simulink model "Sim"  (R2025b)
settings: Solver=FixedStepAuto  StartTime=0.0  StopTime=15724800  FixedStep=300  RelTol=1e-3
values from neighbouring files (symbols this model uses):
  a = 3.5    [Regelung.m]
  b = -0.1    [Regelung.m]
  C = 5.0 * 10^7    (= 50000000)    [Regelung.m]
  eta = 0.20    (= 0.2)    [Regelung.m]
  R = 0.014    [Regelung.m]
settings Model: Creator=Mrhkf  LastModifiedBy=Mrhkf

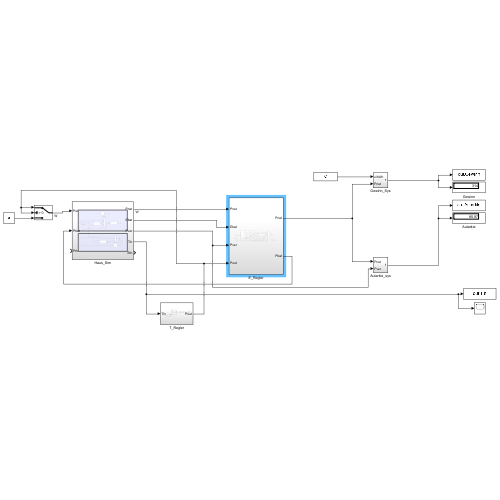
[thumbnail: Simulink's stored preview of the top-level diagram]
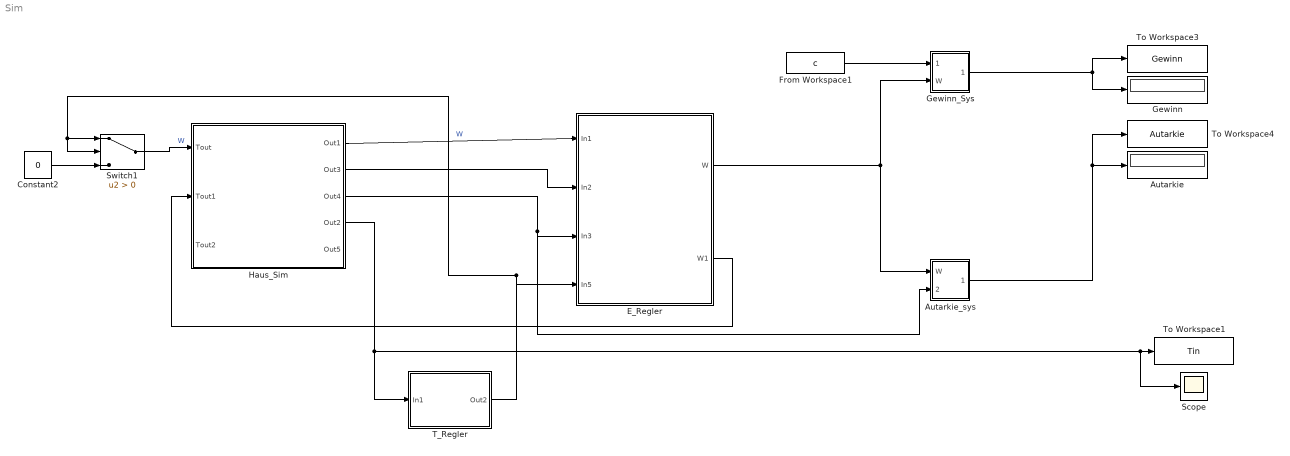
== system Sim ==
  Autarkie : Display
  Autarkie_sys : Subsystem
  Constant2 : Constant  Value=0
  E_Regler : Subsystem
  From Workspace1 : FromWorkspace  VariableName=c  SampleTime=-1  Interpolate=off  OutputAfterFinalValue=Holding final value
  Gewinn : Display
  Gewinn_Sys : Subsystem
  Haus_Sim : Subsystem
  Scope : Scope
      settings: ActiveDisplayYMinimum=17.325726119356677  ActiveDisplayYMaximum=22.113647259135355  DataLoggingVariableName=ScopeData8
  Switch1 : Switch  Criteria=u2 > Threshold  SaturateOnIntegerOverflow=off  InputSameDT=off
  T_Regler : Subsystem
  To Workspace1 : ToWorkspace  VariableName=Tin  SaveFormat=Timeseries  SampleTime=-1
  To Workspace3 : ToWorkspace  VariableName=Gewinn  SaveFormat=Timeseries  SampleTime=-1
  To Workspace4 : ToWorkspace  VariableName=Autarkie  SaveFormat=Timeseries  SampleTime=-1
  wires:
  Switch1/1 -> Haus_Sim/1(Tout)  "W"
  Constant2/1 -> Switch1/3
  Autarkie_sys/1(Out1) -> Autarkie/1, To Workspace4/1
  Gewinn_Sys/1(Out1) -> To Workspace3/1, Gewinn/1
  T_Regler/1(Out2) -> E_Regler/4(In5), Switch1/2, Switch1/1
  Haus_Sim/4(Out2) -> T_Regler/1(In1), Scope/1, To Workspace1/1
  Haus_Sim/3(Out4) -> Autarkie_sys/2(In2), E_Regler/3(In3)
  Haus_Sim/2(Out3) -> E_Regler/2(In2)
  Haus_Sim/1(Out1) -> E_Regler/1(In1)  "W"
  E_Regler/1(W) -> Gewinn_Sys/2(W), Autarkie_sys/1(W)
  From Workspace1/1 -> Gewinn_Sys/1(W1)
  E_Regler/2(W1) -> Haus_Sim/2(Tout1)

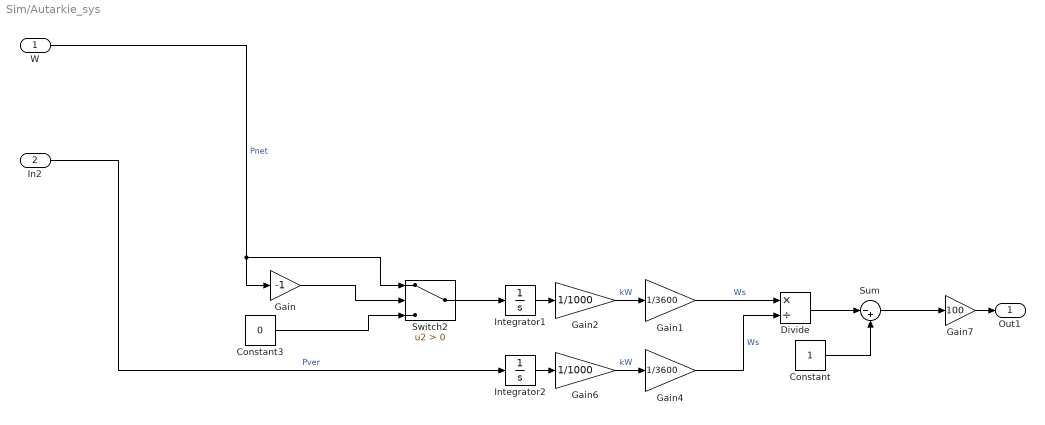
== system Sim/Autarkie_sys ==
  W : Inport
  In2 : Inport  Port=2
  Constant : Constant
  Constant3 : Constant  Value=0
  Divide : Product  Inputs=*/
  Gain : Gain  Gain=-1
  Gain1 : Gain  Gain=1/3600
  Gain2 : Gain  Gain=1/1000
  Gain4 : Gain  Gain=1/3600
  Gain6 : Gain  Gain=1/1000
  Gain7 : Gain  Gain=100
  Integrator1 : Integrator
  Integrator2 : Integrator
  Sum : Sum  Inputs=|-+
  Switch2 : Switch  Criteria=u2 > Threshold  SaturateOnIntegerOverflow=off  InputSameDT=off
  Out1 : Outport
  wires:
  Divide/1 -> Sum/1
  Switch2/1 -> Integrator1/1
  Integrator2/1 -> Gain6/1
  W/1 -> Gain/1, Switch2/1  "Pnet"
  Gain2/1 -> Gain1/1  "kW"
  Gain4/1 -> Divide/2  "Ws"
  Gain1/1 -> Divide/1  "Ws"
  Constant/1 -> Sum/2
  Integrator1/1 -> Gain2/1
  Sum/1 -> Gain7/1
  Gain6/1 -> Gain4/1  "kW"
  Constant3/1 -> Switch2/3
  Gain/1 -> Switch2/2
  Gain7/1 -> Out1/1
  In2/1 -> Integrator2/1  "Pver"

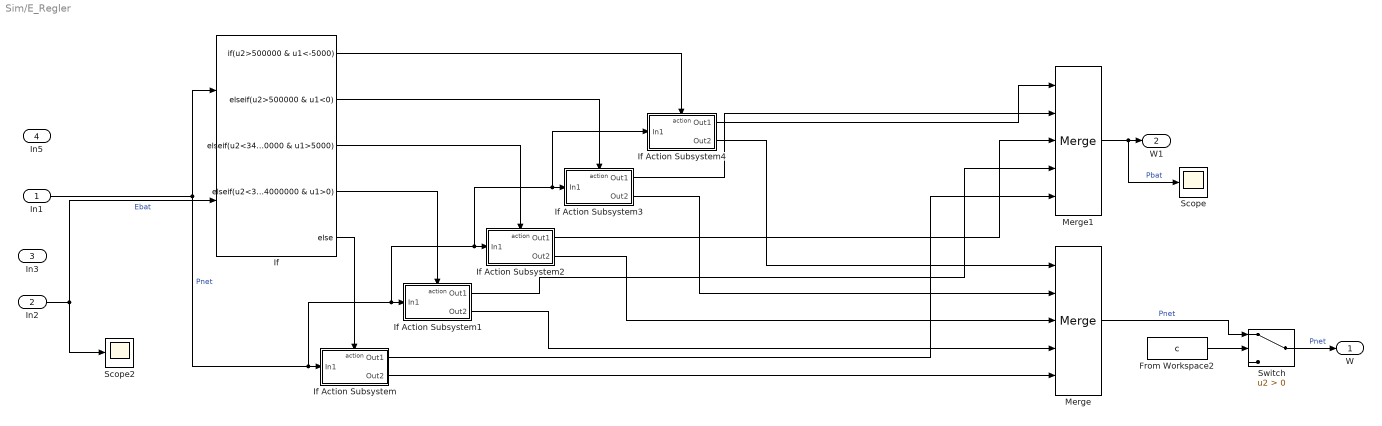
== system Sim/E_Regler ==
  In1 : Inport
  In2 : Inport  Port=2
  In3 : Inport  Port=3
  In5 : Inport  Port=4
  From Workspace2 : FromWorkspace  VariableName=c  SampleTime=-1  Interpolate=off  OutputAfterFinalValue=Holding final value
  If : If  NumInputs=2  IfExpression=u2>500000 & u1<-5000  ElseIfExpressions=u2>500000 & u1<0,u2<34000000 & u1>5000,u2<34000000 & u1>0
  If Action Subsystem : Subsystem  TreatAsAtomicUnit=on
  If Action Subsystem1 : Subsystem  TreatAsAtomicUnit=on
  If Action Subsystem2 : Subsystem  TreatAsAtomicUnit=on
  If Action Subsystem3 : Subsystem  TreatAsAtomicUnit=on
  If Action Subsystem4 : Subsystem  TreatAsAtomicUnit=on
  Merge : Merge  Inputs=5
  Merge1 : Merge  Inputs=5
  Scope : Scope
      settings: ActiveDisplayYMinimum=-8250.3550931605241  ActiveDisplayYMaximum=7676.6931953533167
  Scope2 : Scope
      settings: ActiveDisplayYMinimum=-4.4929612423280012E+6  ActiveDisplayYMaximum=3.9935474879541315E+7  DataLoggingVariableName=ScopeData7
  Switch : Switch  Criteria=u2 > Threshold  SaturateOnIntegerOverflow=off  InputSameDT=off
  W : Outport
  W1 : Outport  Port=2
  wires:
  In1/1 -> If/1, If Action Subsystem1/1(In1), If Action Subsystem2/1(In1), If Action Subsystem4/1(In1), If Action Subsystem3/1(In1), If Action Subsystem/1(In1)  "Pnet"
  In2/1 -> If/2, Scope2/1  "Ebat"
  If/5 -> If Action Subsystem/Action
  If Action Subsystem/2(Out2) -> Merge/5
  If Action Subsystem1/2(Out2) -> Merge/4
  If Action Subsystem2/2(Out2) -> Merge/3
  If Action Subsystem3/2(Out2) -> Merge/2
  If Action Subsystem4/2(Out2) -> Merge/1
  Merge1/1 -> Scope/1, W1/1  "Pbat"
  If Action Subsystem4/1(Out1) -> Merge1/1
  If Action Subsystem3/1(Out1) -> Merge1/2
  If Action Subsystem2/1(Out1) -> Merge1/3
  If Action Subsystem1/1(Out1) -> Merge1/4
  If Action Subsystem/1(Out1) -> Merge1/5
  If/1 -> If Action Subsystem4/Action
  If/2 -> If Action Subsystem3/Action
  If/3 -> If Action Subsystem2/Action
  If/4 -> If Action Subsystem1/Action
  From Workspace2/1 -> Switch/2
  Switch/1 -> W/1  "Pnet"
  Merge/1 -> Switch/1  "Pnet"

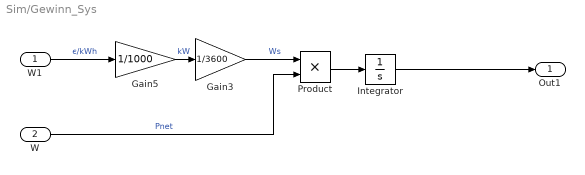
== system Sim/Gewinn_Sys ==
  W1 : Inport
  W : Inport  Port=2
  Gain3 : Gain  Gain=1/3600
  Gain5 : Gain  Gain=1/1000
  Integrator : Integrator
  Product : Product
  Out1 : Outport
  wires:
  W/1 -> Product/2  "Pnet"
  Gain5/1 -> Gain3/1  "kW"
  Product/1 -> Integrator/1
  Gain3/1 -> Product/1  "Ws"
  W1/1 -> Gain5/1  "є/kWh"
  Integrator/1 -> Out1/1

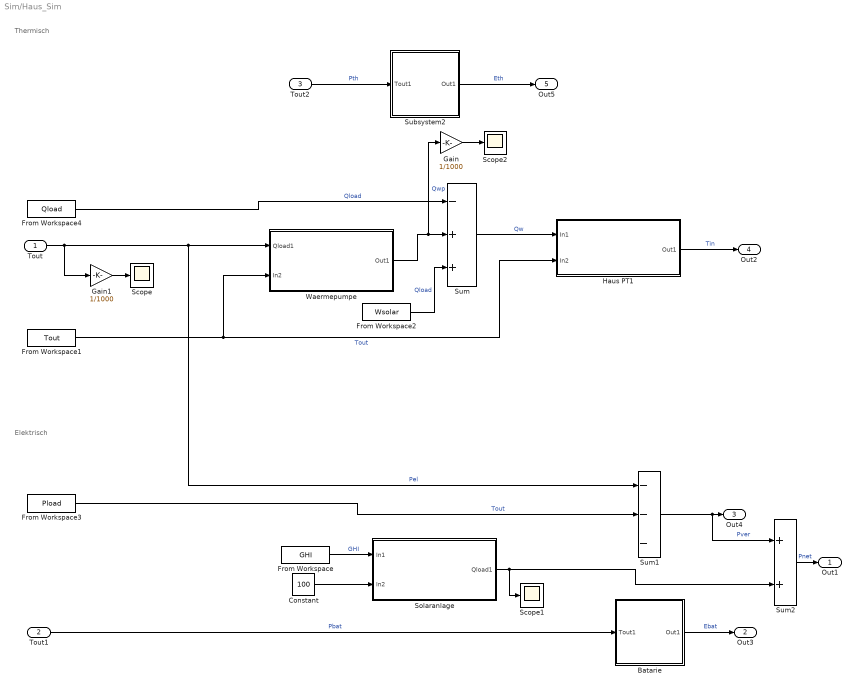
== system Sim/Haus_Sim ==
  note: Thermisch
  note: Elektrisch
  Tout : Inport
  Tout1 : Inport  Port=2
  Tout2 : Inport  Port=3
  Batarie : Subsystem
  Constant : Constant  Value=100
  From Workspace : FromWorkspace  VariableName=GHI  SampleTime=-1  Interpolate=off  OutputAfterFinalValue=Holding final value
  From Workspace1 : FromWorkspace  VariableName=Tout  OutDataTypeStr=double  SampleTime=-1  Interpolate=off  OutputAfterFinalValue=Holding final value
  From Workspace2 : FromWorkspace  VariableName=Wsolar  OutDataTypeStr=double  SampleTime=-1  Interpolate=off  OutputAfterFinalValue=Holding final value
  From Workspace3 : FromWorkspace  VariableName=Pload  SampleTime=-1  Interpolate=off  OutputAfterFinalValue=Holding final value
  From Workspace4 : FromWorkspace  VariableName=Qload  OutDataTypeStr=double  SampleTime=-1  Interpolate=off  OutputAfterFinalValue=Holding final value
  Gain : Gain  Gain=1/1000
  Gain1 : Gain  Gain=1/1000
  Haus PT1 : Subsystem  Description=fsfsf
  Scope : Scope
      settings: ActiveDisplayYMinimum=-0.21662082419067072  ActiveDisplayYMaximum=1.9495874177160371
  Scope1 : Scope
      settings: ActiveDisplayYMinimum=-2299.9999999999995  ActiveDisplayYMaximum=20700  DataLoggingVariableName=ScopeData5
  Scope2 : Scope
      settings: ActiveDisplayYMinimum=-1.0190071272282573  ActiveDisplayYMaximum=9.1710641450543164  DataLoggingVariableName=ScopeData6
  "Solaranlage " : Subsystem
  Subsystem2 : Subsystem
  Sum : Sum  Inputs=-++
  Sum1 : Sum  Inputs=---
  Sum2 : Sum
  Waermepumpe : Subsystem
  Out1 : Outport
  Out3 : Outport  Port=2
  Out4 : Outport  Port=3
  Out2 : Outport  Port=4
  Out5 : Outport  Port=5
  wires:
  Constant/1 -> "Solaranlage "/2(In2)
  From Workspace3/1 -> Sum1/2  "Tout"
  Batarie/1(Out1) -> Out3/1  "Ebat"
  From Workspace1/1 -> Waermepumpe/2(In2), Haus PT1/2(In2)  "Tout"
  Waermepumpe/1(Out1) -> Gain/1, Sum/2  "Qwp"
  Tout1/1 -> Batarie/1(Tout1)  "Pbat"
  Haus PT1/1(Out1) -> Out2/1  "Tin"
  From Workspace/1 -> "Solaranlage "/1(In1)  "GHI"
  Sum/1 -> Haus PT1/1(In1)  "Qw"
  Tout/1 -> Gain1/1, Sum1/1, Waermepumpe/1(Qload1)  "Pel"
  Sum1/1 -> Sum2/1, Out4/1  "Pver"
  "Solaranlage "/1(Qload1) -> Scope1/1, Sum2/2
  Sum2/1 -> Out1/1  "Pnet"
  From Workspace2/1 -> Sum/3  "Qload"
  Subsystem2/1(Out1) -> Out5/1  "Eth"
  Tout2/1 -> Subsystem2/1(Tout1)  "Pth"
  From Workspace4/1 -> Sum/1  "Qload"
  Gain/1 -> Scope2/1
  Gain1/1 -> Scope/1

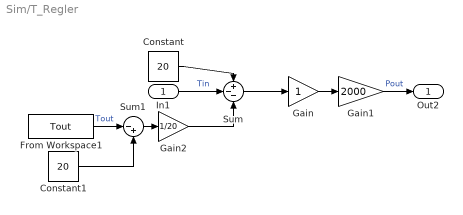
== system Sim/T_Regler ==
  In1 : Inport
  Constant : Constant  Value=20
  Constant1 : Constant  Value=20
  From Workspace1 : FromWorkspace  VariableName=Tout  OutDataTypeStr=double  SampleTime=-1  Interpolate=off  OutputAfterFinalValue=Holding final value
  Gain : Gain
  Gain1 : Gain  Gain=2000
  Gain2 : Gain  Gain=1/20
  Sum : Sum  Inputs=+--
  Sum1 : Sum  Inputs=|-+
  Out2 : Outport
  wires:
  Constant/1 -> Sum/1
  In1/1 -> Sum/2  "Tin"
  Sum/1 -> Gain/1
  Gain/1 -> Gain1/1
  From Workspace1/1 -> Sum1/1  "Tout"
  Constant1/1 -> Sum1/2
  Gain1/1 -> Out2/1  "Pout"
  Sum1/1 -> Gain2/1
  Gain2/1 -> Sum/3

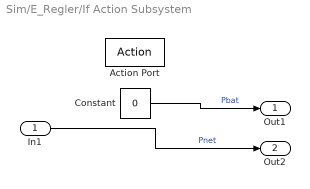
== system Sim/E_Regler/If Action Subsystem ==
  In1 : Inport
  Action Port : ActionPort  ActionPortLabel=else
  Constant : Constant  Value=0
  Out1 : Outport
  Out2 : Outport  Port=2
  wires:
  In1/1 -> Out2/1  "Pnet"
  Constant/1 -> Out1/1  "Pbat"

== system Sim/E_Regler/If Action Subsystem1 ==
  In1 : Inport
  Action Port : ActionPort  ActionPortLabel=elseif(u2<34000000 & u1>0)
  Constant : Constant  Value=0
  Out1 : Outport
  Out2 : Outport  Port=2
  wires:
  Constant/1 -> Out2/1  "Pnet"
  In1/1 -> Out1/1  "Pbat"

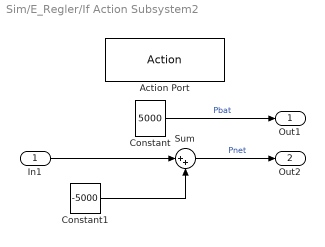
== system Sim/E_Regler/If Action Subsystem2 ==
  In1 : Inport
  Action Port : ActionPort  ActionPortLabel=elseif(u2<34000000 & u1>5000)
  Constant : Constant  Value=5000
  Constant1 : Constant  Value=-5000
  Sum : Sum  Inputs=|++
  Out1 : Outport
  Out2 : Outport  Port=2
  wires:
  Sum/1 -> Out2/1  "Pnet"
  Constant/1 -> Out1/1  "Pbat"
  In1/1 -> Sum/1
  Constant1/1 -> Sum/2

== system Sim/E_Regler/If Action Subsystem3 ==
  In1 : Inport
  Action Port : ActionPort  ActionPortLabel=elseif(u2>500000 & u1<0)
  Constant : Constant  Value=0
  Out1 : Outport
  Out2 : Outport  Port=2
  wires:
  Constant/1 -> Out2/1  "Pnet"
  In1/1 -> Out1/1  "Pbat"

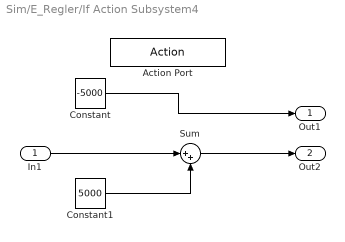
== system Sim/E_Regler/If Action Subsystem4 ==
  In1 : Inport
  Action Port : ActionPort  ActionPortLabel=if(u2>500000 & u1<-5000)
  Constant : Constant  Value=-5000
  Constant1 : Constant  Value=5000
  Sum : Sum  Inputs=|++
  Out1 : Outport
  Out2 : Outport  Port=2
  wires:
  Constant/1 -> Out1/1
  In1/1 -> Sum/1
  Sum/1 -> Out2/1
  Constant1/1 -> Sum/2

== system Sim/Haus_Sim/Batarie ==
  Tout1 : Inport
  Integrator : Integrator  InitialCondition=5*1000*3600
  Out1 : Outport
  wires:
  Integrator/1 -> Out1/1  "Ebat"
  Tout1/1 -> Integrator/1  "Pbat"

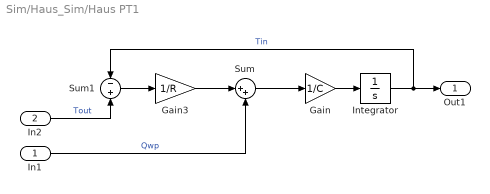
== system Sim/Haus_Sim/Haus PT1 ==
  In1 : Inport
  In2 : Inport  Port=2
  Gain : Gain  Gain=1/C
  Gain3 : Gain  Gain=1/R
  Integrator : Integrator  InitialCondition=20
  Sum : Sum  Inputs=|++
  Sum1 : Sum  Inputs=-+
  Out1 : Outport
  wires:
  In1/1 -> Sum/2  "Qwp"
  Sum1/1 -> Gain3/1
  Gain/1 -> Integrator/1
  Sum/1 -> Gain/1
  Integrator/1 -> Sum1/1, Out1/1  "Tin"
  Gain3/1 -> Sum/1
  In2/1 -> Sum1/2  "Tout"

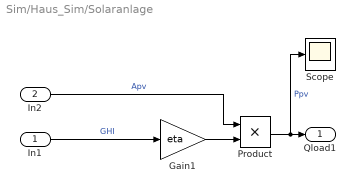
== system Sim/Haus_Sim/Solaranlage  ==
  In1 : Inport
  In2 : Inport  Port=2
  Gain1 : Gain  Gain=eta
  Product : Product
  Scope : Scope
      settings: ActiveDisplayYMinimum=-2299.9999999999995  ActiveDisplayYMaximum=20700  DataLoggingVariableName=ScopeData2
  Qload1 : Outport
  wires:
  In1/1 -> Gain1/1  "GHI"
  Gain1/1 -> Product/2
  Product/1 -> Scope/1, Qload1/1  "Ppv"
  In2/1 -> Product/1  "Apv"

== system Sim/Haus_Sim/Subsystem2 ==
  Tout1 : Inport
  Integrator : Integrator  InitialCondition=3.5*1000*3600
  Out1 : Outport
  wires:
  Integrator/1 -> Out1/1  "Ebat"
  Tout1/1 -> Integrator/1  "Pbat"

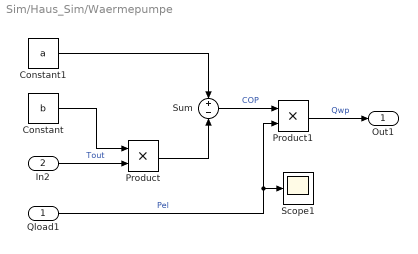
== system Sim/Haus_Sim/Waermepumpe ==
  Qload1 : Inport
  In2 : Inport  Port=2
  Constant : Constant  Value=b
  Constant1 : Constant  Value=a
  Product : Product
  Product1 : Product
  Scope1 : Scope
      settings: ActiveDisplayYMinimum=-3425.2311606918129  ActiveDisplayYMaximum=7155.8608944907819  DataLoggingVariableName=ScopeData4
  Sum : Sum  Inputs=+-
  Out1 : Outport
  wires:
  Constant1/1 -> Sum/1
  Constant/1 -> Product/1
  In2/1 -> Product/2  "Tout"
  Product/1 -> Sum/2
  Sum/1 -> Product1/1  "COP"
  Qload1/1 -> Scope1/1, Product1/2  "Pel"
  Product1/1 -> Out1/1  "Qwp"
